simulink model "kinematic_arm_simulation"  (Simulink 8.3)
settings: Solver=FixedStepDiscrete  SolverMode=SingleTasking  StartTime=0.0  StopTime=50  FixedStep=.01  RelTol=1e-3  AbsTol=1e-6
undefined symbols (not defined in the file or in its folder): DiscIntNeverNeededParam, forward_kinematics, inverse_kinematics
libraries: simulink x1
settings Model: Creator=sschaal  LastModifiedBy=Bob  ExtModeAutoUpdateStatusClock=off
settings DataIOCC: LimitDataPoints=off  SaveOutput=off
settings OptimizationCC: BlockReduction=off  BooleanDataType=off  ExpressionDepthLimit=2147483647  InitFltsAndDblsToZero=on
settings DebuggingCC: SaveWithParameterizedLinksMsg=none  SignalResolutionControl=TryResolveAllWithWarning  SolverPrmCheckMsg=none  MultiTaskDSMMsg=warning  MultiTaskCondExecSysMsg=none  FcnCallInpInsideContextMsg=UseLocalSettings
settings HardwareCC: TargetUnknown=on
settings RTWCC: IncludeERTFirstTime=on
settings GRTTargetCC: TargetFcnLib=ansi_tfl_tmw.mat

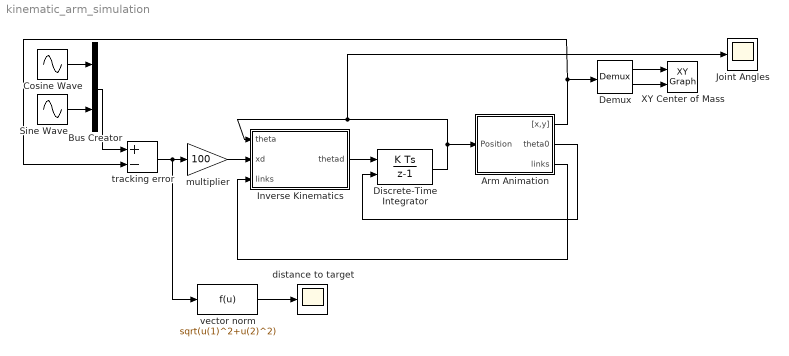
== system kinematic_arm_simulation ==
  Arm Animation : Subsystem  mask(ArmAnimation){links=[0.3 0.15 0.2 0.05], theta0=[-0.4302;0.149;0.3393; 0.4422], ts=.05}
      mask prompts: links "Link Lengths"; theta0 "Initial Posture"; ts "Sample time:"
  Bus Creator : BusCreator  Inputs=2
  Cosine Wave : Sin  Amplitude=.15  Bias=0.2  Frequency=pi/5  Phase=pi/2  SampleTime=0
  Demux : Demux  Outputs=2
  Discrete-Time Integrator : DiscreteIntegrator  InitialConditionSource=external  SampleTime=0.01  ICPrevOutput=DiscIntNeverNeededParam  ICPrevScaledInput=DiscIntNeverNeededParam
  Inverse Kinematics : Subsystem  mask(Inverse Kinematics){}
  Joint Angles : Scope
      settings: YMin=-2.5  YMax=17.5
  Sine Wave : Sin  Amplitude=.15  Frequency=pi/5  SampleTime=0
  XY Center of Mass : simulink/Sinks/XY Graph  xmin=-.5  xmax=.5  ymin=-.5  ymax=.5  st=-1
  distance to target : Scope
      settings: TickLabels=on  YMin=0.05  YMax=0.4
  multiplier : Gain  Gain=100  SaturateOnIntegerOverflow=on  OutDataTypeStr=Inherit: Same as input  ParamDataTypeStr=Inherit: Same as input
  tracking error : Sum  Inputs=+-  SaturateOnIntegerOverflow=on  InputSameDT=on  OutDataTypeStr=Inherit: Same as first input
  vector norm : Fcn  Expr=sqrt(u(1)^2+u(2)^2)
  wires:
  multiplier/1 -> Inverse Kinematics/2(xd)
  Inverse Kinematics/1(thetad) -> Discrete-Time Integrator/1
  Discrete-Time Integrator/1 -> Arm Animation/1(Position), Inverse Kinematics/1(theta), Joint Angles/1
  Demux/1 -> XY Center of Mass/1
  Demux/2 -> XY Center of Mass/2
  Arm Animation/3(links) -> Inverse Kinematics/3(links)
  Arm Animation/2(theta0) -> Discrete-Time Integrator/2
  Arm Animation/1("[x,y]") -> Demux/1, tracking error/2
  tracking error/1 -> multiplier/1, vector norm/1
  vector norm/1 -> distance to target/1
  Bus Creator/1 -> tracking error/1
  Cosine Wave/1 -> Bus Creator/1
  Sine Wave/1 -> Bus Creator/2

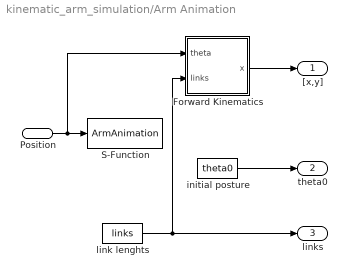
== system kinematic_arm_simulation/Arm Animation ==
  Position : Inport
  Forward Kinematics : Subsystem  mask(Forward Kinematics){}
  S-Function : S-Function  FunctionName=ArmAnimation  Parameters=ts,theta0,links  EnableBusSupport=off
  initial posture : Constant  Value=theta0
  link lenghts : Constant  Value=links
  "[x,y]" : Outport
  theta0 : Outport  Port=2
  links : Outport  Port=3
  wires:
  initial posture/1 -> theta0/1
  Position/1 -> S-Function/1, Forward Kinematics/1(theta)
  Forward Kinematics/1(x) -> "[x,y]"/1
  link lenghts/1 -> links/1, Forward Kinematics/2(links)

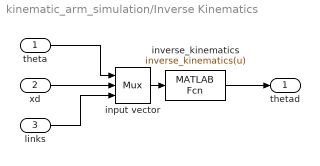
== system kinematic_arm_simulation/Inverse Kinematics ==
  theta : Inport
  xd : Inport  Port=2
  links : Inport  Port=3
  input vector : Mux  Inputs=3
  inverse_kinematics : MATLABFcn  MATLABFcn=inverse_kinematics(u)
  thetad : Outport  InitialOutput=0
  wires:
  theta/1 -> input vector/1
  xd/1 -> input vector/2
  input vector/1 -> inverse_kinematics/1
  links/1 -> input vector/3
  inverse_kinematics/1 -> thetad/1

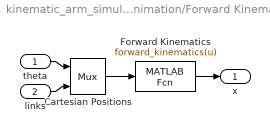
== system kinematic_arm_simulation/Arm Animation/Forward Kinematics ==
  theta : Inport
  links : Inport  Port=2
  Cartesian Positions : Mux  Inputs=2
  Forward Kinematics : MATLABFcn  MATLABFcn=forward_kinematics(u)  OutputDimensions=2
  x : Outport  InitialOutput=0
  wires:
  Forward Kinematics/1 -> x/1
  theta/1 -> Cartesian Positions/1
  links/1 -> Cartesian Positions/2
  Cartesian Positions/1 -> Forward Kinematics/1
